simulink model "E_Netzwerk"  (R2017b)
settings: Solver=ode45  StartTime=0.0  StopTime=2  RelTol=1e-3
values from neighbouring files (symbols this model uses):
  A = [A11,A12;A21,A22]    [Esys_Parameter.m]
  B = [bu,bd]    [Esys_Parameter.m]
  C1_ref = 1e-6    (= 1e-06)    [Esys_Parameter.m]    (also in Esys_S_m.m = block.DialogPrm(6).Data)
  C2 = 1e-6    (= 1e-06)    [Esys_Parameter.m]    (also in Esys_S_m.m = block.DialogPrm(9).Data)
  K = 3    [Esys_Parameter.m]    (also in Esys_S_m.m = block.DialogPrm(5).Data)
  kC1 = 800e-9    (= 8e-07)    [Esys_Parameter.m]    (also in Esys_S_m.m = block.DialogPrm(8).Data)
  R1 = 625    [Esys_Parameter.m]    (also in Esys_S_m.m = block.DialogPrm(3).Data)
  R2 = 3500    [Esys_Parameter.m]    (also in Esys_S_m.m = block.DialogPrm(4).Data)
  te = 0.05    [Esys_Parameter.m]
  ts = 0.1    [Esys_Parameter.m]
  UaR = K * UC2R    (= 15)    [Esys_Parameter.m]
  UC1_ref = -10    [Esys_Parameter.m]    (also in Esys_S_m.m = block.DialogPrm(7).Data)
  UC1R = -(K-2)*(R2*UeR+(R1+R2)*UsR)/(R1+2*R2)-UsR    (= -10)    [Esys_Parameter.m]
  UC2R = (R2*UeR+(R1+R2)*UsR)/(R1+2*R2)    (= 5)    [Esys_Parameter.m]
  Ue = 7    [Esys_Parameter.m]    (also in Esys_S_m.m = u(1))
  UeR = 5    [Esys_Parameter.m]
  Us = 4    [Esys_Parameter.m]    (also in Esys_S_m.m = u(2))
  Usinus = 1    [Esys_Parameter.m]
  UsR = 5    [Esys_Parameter.m]
  we = 1000    [Esys_Parameter.m]
libraries: cstblocks x4, simulink x1
settings Model: Creator=sj  LastModifiedBy=user
settings DataIOCC: LimitDataPoints=on  SaveFormat=Array
settings OptimizationCC: BlockReduction=off  BooleanDataType=off  LifeSpan=inf
settings DebuggingCC: SaveWithParameterizedLinksMsg=none  UnderspecifiedInitializationDetection=Classic  MergeDetectMultiDrivingBlocksExec=none  SignalResolutionControl=TryResolveAllWithWarning  SFUnexpectedBacktrackingDiag=warning  SFNoUnconditionalDefaultTransitionDiag=warning  SFExecutionAtInitializationDiag=none
settings HardwareCC: ProdBitPerPointer=32  ProdBitPerSizeT=32  ProdBitPerPtrDiffT=32  ProdLargestAtomicFloat=None  ProdIntDivRoundTo=Undefined  ProdEndianess=Unspecified  ProdWordSize=32  ProdHWDeviceType=32-bit Generic  TargetUnknown=on
settings ModelReferenceCC: PropagateSignalLabelsOutOfModel=off
settings CodeAppCC: StateflowObjectComments=on
settings GRTTargetCC: TargetLangStandard=C89/C90 (ANSI)  GeneratePreprocessorConditionals=Disable all
settings ConfigComp: CovMetricSettings=dw  CovHtmlReporting=on  CovSaveCumulativeToWorkspaceVar=on  CovSaveSingleToWorkspaceVar=on  CovExternalEMLEnable=off  CovSFcnEnable=off

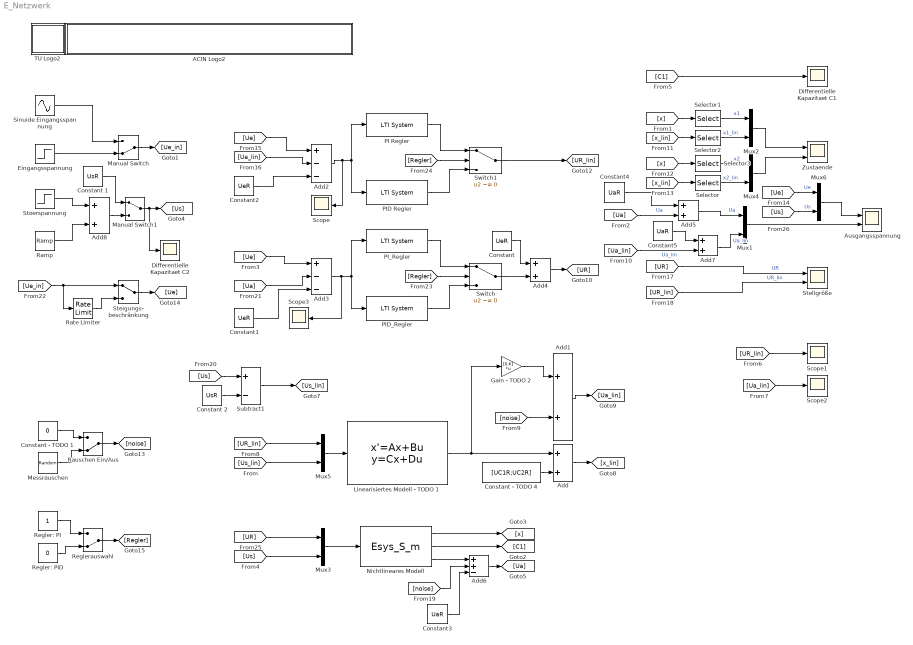
== system E_Netzwerk ==
  ACIN Logo2 : Subsystem
      mask init:
      | s = get_param(gcb,'UserData');
      mask Display:
      | image(s.logo,[0 0 439 45]);
      | %axis image
  Add{,1,5,7..8} (5 alike) : Sum
  Add2 : Sum  Inputs=+--
  Add3 : Sum  Inputs=+--
  Add4 : Sum  CollapseMode=Specified dimension
  Add6 : Sum  Inputs=++-
  Ausgangsspannung : Scope  NumInputPorts=2
  Constant : Constant  Value=UeR
  Constant - TODO 1 : Constant  Value=0
  Constant - TODO 4 : Constant  Value=[UC1R;UC2R]
  Constant 1 : Constant  Value=UsR
  Constant 2 : Constant  Value=UsR
  Constant1 : Constant  Value=UeR
  Constant2 : Constant  Value=UeR
  Constant3 : Constant  Value=UaR
  Constant4 : Constant  Value=UaR
  Constant5 : Constant  Value=UaR
  Differentielle Kapazitaet C1 : Scope
  Differentielle Kapazitaet C2 : Scope
  Eingangsspannung : Step  Time=te  Before=UeR  After=Ue  SampleTime=0
  Gain - TODO 2 : Gain  Gain=[0,K]  Multiplication=Matrix(K*u)
  Linearisiertes Modell - TODO 1 : StateSpace  A=A  B=B  C=[1, 0; 0, 1]  D=[0,0;0,0]  InitialCondition=[0,0]
  Manual Switch : ManualSwitch  CurrentSetting=0
  Manual Switch1 : ManualSwitch
  Messrauschen : UniformRandomNumber  Minimum=-5e-2  Maximum=5e-2  SampleTime=1e-3
  Mux{1..6} (6 alike) : Mux  Inputs=2
  Nichtlineares Modell : M-S-Function  FunctionName=Esys_S_m  Parameters=UC1R,UC2R,R1,R2,K,C1_ref,UC1_ref,kC1,C2
  PI Regler : cstblocks/LTI System  sys=R_pi  IC=[]
  PID Regler : cstblocks/LTI System  sys=R_pid  IC=[]
  PID_Regler : cstblocks/LTI System  sys=R_pid  IC=[]
  PI_Regler : cstblocks/LTI System  sys=R_pi  IC=[]
  Ramp : simulink/Sources/Ramp  slope=1  start=0  X0=0
  Rate Limiter : RateLimiter  RisingSlewLimit=100  FallingSlewLimit=-100  SampleTimeMode=inherited
  Rauschen Ein/Aus : ManualSwitch  CurrentSetting=0
  Regler: PI : Constant
  Regler: PID : Constant  Value=0
  Reglerauswahl : ManualSwitch  CurrentSetting=0
  Scope{,1..3} (4 alike) : Scope
  Selector : Selector  InputPortWidth=2  IndexOptions=Index vector (dialog)  Indices=2  OutputSizes=1
  Selector1 : Selector  InputPortWidth=2  IndexOptions=Index vector (dialog)  Indices=1  OutputSizes=1
  Selector2 : Selector  InputPortWidth=2  IndexOptions=Index vector (dialog)  Indices=1  OutputSizes=1
  Selector3 : Selector  InputPortWidth=2  IndexOptions=Index vector (dialog)  Indices=2  OutputSizes=1
  Sinuide Eingangsspannung : Sin  Amplitude=Usinus  Bias=UeR  Frequency=we  SampleTime=0
  Steigungs- beschränkung : ManualSwitch
  Stellgröße : Scope  NumInputPorts=2
  Stoerspannung : Step  Time=ts  Before=UsR  After=Us  SampleTime=0
  Subtract1 : Sum  Inputs=+-
  Switch : Switch  Criteria=u2 ~= 0
  Switch1 : Switch  Criteria=u2 ~= 0
  TU Logo2 : Subsystem
      mask init:
      | s = get_param(gcb,'UserData');
      mask Display: image(s.logo,[0 0 45 45]);
  Zustaende : Scope  NumInputPorts=2
  wires:
  Nichtlineares Modell/1 -> [x]
  Nichtlineares Modell/2 -> [C1]
  Eingangsspannung/1 -> Manual Switch/2
  Sinuide Eingangsspannung/1 -> Manual Switch/1
  Manual Switch/1 -> [Ue_in]
  [C1] -> Differentielle Kapazitaet C1/1
  Selector1/1 -> Mux2/1  "x1"
  Selector2/1 -> Mux2/2  "x1_lin"
  [x] -> Selector1/1
  [x_lin] -> Selector2/1
  Selector3/1 -> Mux4/1  "x2"
  Selector/1 -> Mux4/2  "x2_lin"
  [x] -> Selector3/1
  [x_lin] -> Selector/1
  Mux2/1 -> Zustaende/1
  Mux4/1 -> Zustaende/2
  [UR] -> Stellgröße/1  "UR"
  [UR_lin] -> Stellgröße/2  "UR_lin"
  Add3/1 -> Scope3/1, PI_Regler/1, PID_Regler/1
  Mux3/1 -> Nichtlineares Modell/1
  Messrauschen/1 -> Rauschen Ein/Aus/2
  Constant - TODO 1/1 -> Rauschen Ein/Aus/1
  Rauschen Ein/Aus/1 -> [noise]
  Add6/1 -> [Ua]
  Nichtlineares Modell/3 -> Add6/1
  [noise] -> Add6/2
  Steigungs- beschränkung/1 -> [Ue]
  [Ue_in] -> Rate Limiter/1, Steigungs- beschränkung/1
  Rate Limiter/1 -> Steigungs- beschränkung/2
  PI_Regler/1 -> Switch/1
  [Regler] -> Switch/2
  Regler: PID/1 -> Reglerauswahl/2
  Regler: PI/1 -> Reglerauswahl/1
  Reglerauswahl/1 -> [Regler]
  PID_Regler/1 -> Switch/3
  PI Regler/1 -> Switch1/1
  [Regler] -> Switch1/2
  PID Regler/1 -> Switch1/3
  Switch1/1 -> [UR_lin]
  Stoerspannung/1 -> Add8/1
  Ramp/1 -> Add8/2
  Add2/1 -> Scope/1, PID Regler/1, PI Regler/1
  Add1/1 -> [Ua_lin]
  Mux5/1 -> Linearisiertes Modell - TODO 1/1
  Gain - TODO 2/1 -> Add1/1
  Linearisiertes Modell - TODO 1/1 -> Gain - TODO 2/1, Add/1
  Constant - TODO 4/1 -> Add/2
  Add/1 -> [x_lin]
  [Ue] -> Add2/1
  [Ua_lin] -> Add2/2
  [UR_lin] -> Mux5/1
  [Us_lin] -> Mux5/2
  [UR_lin] -> Scope1/1
  [Ua_lin] -> Scope2/1
  [Ua] -> Add3/2
  [Ue] -> Add3/1
  Add4/1 -> [UR]
  Switch/1 -> Add4/2
  Constant/1 -> Add4/1
  [Us] -> Subtract1/1
  Subtract1/1 -> [Us_lin]
  Constant 2/1 -> Subtract1/2
  [UR] -> Mux3/1
  [Us] -> Mux3/2
  Add8/1 -> Manual Switch1/2
  Manual Switch1/1 -> Differentielle Kapazitaet C2/1, [Us]
  Mux1/1 -> Ausgangsspannung/2
  [Ue] -> Mux6/1  "Ue"
  Mux6/1 -> Ausgangsspannung/1
  [Us] -> Mux6/2  "Us"
  Constant 1/1 -> Manual Switch1/1
  Constant1/1 -> Add3/3
  Constant2/1 -> Add2/3
  Constant3/1 -> Add6/3
  [Ua] -> Add5/2  "Ua"
  Add5/1 -> Mux1/1  "Ua"
  Constant4/1 -> Add5/1
  [Ua_lin] -> Add7/2  "Ua_lin"
  Constant5/1 -> Add7/1
  Add7/1 -> Mux1/2  "Ua_lin"
  [noise] -> Add1/2

== system E_Netzwerk/ACIN Logo2 ==

== system E_Netzwerk/TU Logo2 ==
